simulink model "esercizio1"  (Simulink 8.5)
settings: Solver=ode45  StartTime=0.0  StopTime=10  RelTol=1e-3
libraries: simulink x4
settings Model: Creator=DOC_CS31  LastModifiedBy=Alessandra
settings OptimizationCC: InitFltsAndDblsToZero=on
settings DebuggingCC: SaveWithParameterizedLinksMsg=none  SolverPrmCheckMsg=warning  FcnCallInpInsideContextMsg=UseLocalSettings
settings GRTTargetCC: TargetFcnLib=ansi_tfl_tmw.mat

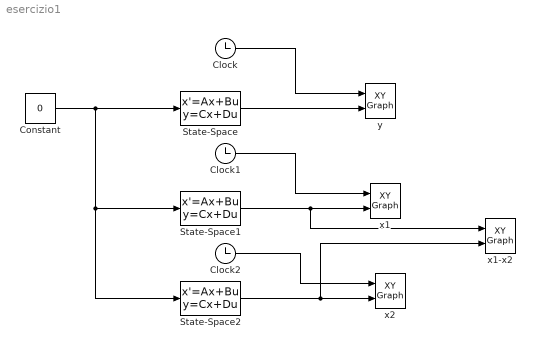
== system esercizio1 ==
  Clock : Clock
  Clock1 : Clock
  Clock2 : Clock
  Constant : Constant  Value=0
  State-Space : StateSpace  A=[-1 -10;10 -1]  B=[1 2]'  C=[1 -1]  D=0  X0=[1 1]'
  State-Space1 : StateSpace  A=[-1 -10;10 -1]  B=[1 2]'  C=[1 0]  D=0  X0=[1 1]'
  State-Space2 : StateSpace  A=[-1 -10;10 -1]  B=[1 2]'  C=[0 1]  D=0  X0=[1 1]'
  x1 : simulink/Sinks/XY Graph  xmin=0  xmax=10  ymin=-1.5  ymax=1.5  st=0.01
  x1-x2 : simulink/Sinks/XY Graph  xmin=-1.5  xmax=1.5  ymin=-1.5  ymax=1.5  st=0.01
  x2 : simulink/Sinks/XY Graph  xmin=0  xmax=10  ymin=-1.5  ymax=1.5  st=0.01
  y : simulink/Sinks/XY Graph  xmin=0  xmax=10  ymin=-2.2  ymax=2  st=0.01
  wires:
  Constant/1 -> State-Space1/1, State-Space2/1, State-Space/1
  Clock/1 -> y/1
  State-Space/1 -> y/2
  Clock1/1 -> x1/1
  State-Space1/1 -> x1/2, x1-x2/1
  Clock2/1 -> x2/1
  State-Space2/1 -> x2/2, x1-x2/2
